simulink model "DNN_Final_Model"  (R2023a)
settings: Solver=VariableStepAuto  StartTime=0.0  StopTime=30  RelTol=1e-3
undefined symbols (not defined in the file or in its folder): c1, K1, k1, k2, m1, m2
libraries: simulink x5, spsVoltageMeasurementLib x3, slpidlib x2, eeGeneralControl x1, spsUniversalBridgeLib x1, spsDCVoltageSourceLib x1, sps_lib x1
settings Model: Creator=liu  LastModifiedBy=Probook
settings SolverCC: AlgebraicLoopSolver=TrustRegion
settings DataIOCC: ReturnWorkspaceOutputs=off
settings DebuggingCC: UnconnectedInputMsg=warning  UnconnectedOutputMsg=warning  UnconnectedLineMsg=warning  ArithmeticOperatorsInVariantConditions=warning
settings ModelReferenceCC: EnableRefExpFcnMdlSchedulingChecks=on
settings SFSimCC: CustomCodeUndefinedFunction=UseInterfaceOnly

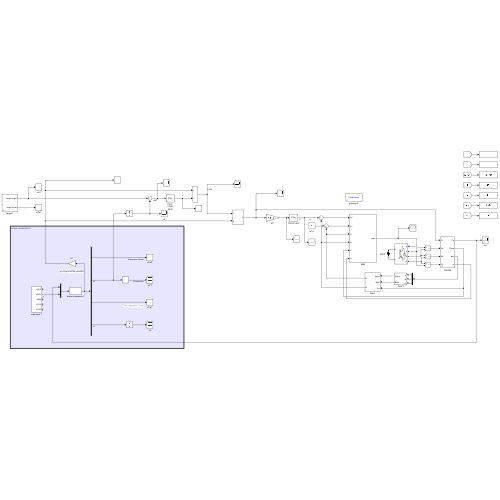
[thumbnail: Simulink's stored preview of the top-level diagram]
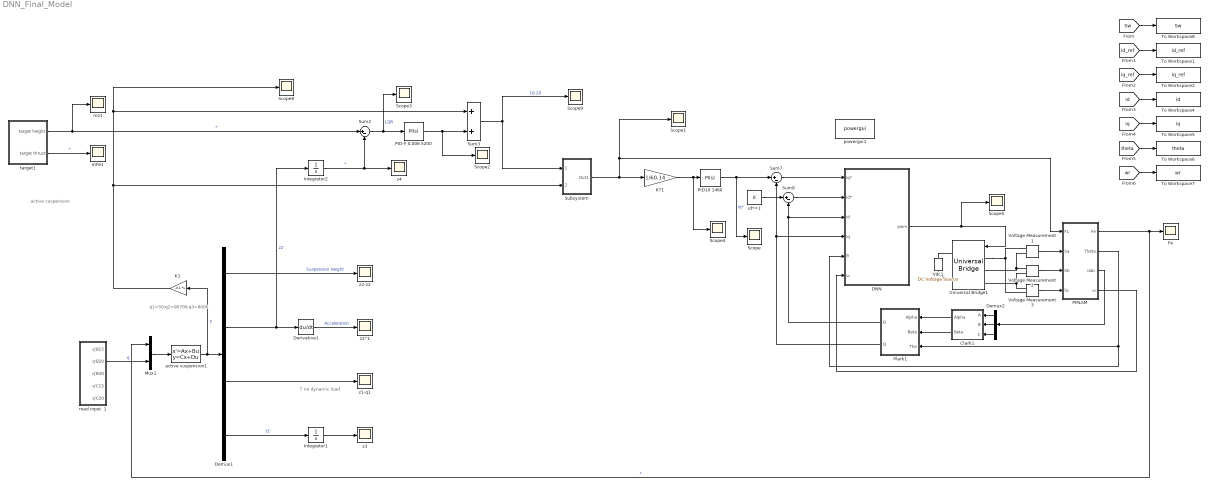
== system DNN_Final_Model ==
  note: T ire dynamic load
  note: active suspension
  note: q1=50;q2=90700;q3=8000
  Clark1 : Subsystem
  DNN : Subsystem
  Demux1 : Demux
  Demux2 : Demux  Outputs=3
  Derivative1 : Derivative
  Fe : Scope
  Integrator1 : Integrator
  Integrator2 : Integrator
  K1 : Gain  Gain=-K1  Multiplication=Matrix(K*u)
  KT1 : Gain  Gain=1/60.14
  Mux1 : Mux  Inputs=2
  PID-F 0.006 5200 : slpidlib/PID Controller  Controller=PI  Form=Parallel  TimeDomain=Continuous-time  UseExternalTs=off  SampleTime=-1  IntegratorMethod=Forward Euler  FilterMethod=Forward Euler  ControllerParametersSource=internal  P=0.006  I=62000  UseKiTs=off  D=10  N=100  UseFilter=on  TunerSelectOption=Transfer Function Based (PID Tuner App)  InitialConditionSource=internal  InitialConditionForIntegrator=0  InitialConditionForFilter=0  DifferentiatorICPrevScaledInput=0  ExternalReset=none  TrackingMode=off  Kt=1  LimitOutput=off  SatLimitsSource=internal  UpperSaturationLimit=inf  LowerSaturationLimit=-inf  LinearizeAsGain=on  AntiWindupMode=none  Kb=1  LimitIntegrator=off  UpperIntegratorSaturationLimit=inf  LowerIntegratorSaturationLimit=-inf  POutMin=[]  POutMax=[]  IOutMin=[]  IOutMax=[]  DOutMin=[]  DOutMax=[]  NOutMin=[]  NOutMax=[]  SumOutMin=[]  SumOutMax=[]  SaturationOutMin=[]  SaturationOutMax=[]  PParamMin=[]  PParamMax=[]  IParamMin=[]  IParamMax=[]  DParamMin=[]  DParamMax=[]  NParamMin=[]  NParamMax=[]  KbParamMin=[]  KbParamMax=[]  KtParamMin=[]  KtParamMax=[]  KbOutMin=[]  KbOutMax=[]  KtOutMin=[]  KtOutMax=[]  IntegratorOutMin=[]  IntegratorOutMax=[]  FilterOutMin=[]  FilterOutMax=[]  SumI1OutMin=[]  SumI1OutMax=[]  SumI2OutMin=[]  SumI2OutMax=[]  SumI3OutMin=[]  SumI3OutMax=[]  SumI4OutMin=[]  SumI4OutMax=[]  SumDOutMin=[]  SumDOutMax=[]  DifferentiatorOutMin=[]  DifferentiatorOutMax=[]  FilterDiffOutCoefMin=[]  FilterDiffOutCoefMax=[]  ReciprocalOutMin=[]  ReciprocalOutMax=[]  SumDenOutMin=[]  SumDenOutMax=[]  SumNumOutMin=[]  SumNumOutMax=[]  DivideOutMin=[]  DivideOutMax=[]  UdiffTsProdOutMin=[]  UdiffTsProdOutMax=[]  NTsProdOutMin=[]  NTsProdOutMax=[]  UintegralTsProdOutMin=[]  UintegralTsProdOutMax=[]  UngainTsProdOutMin=[]  UngainTsProdOutMax=[]  ClampingZeroOutDataTypeStr=Inherit: Inherit via back propagation  ClampingZeroOutMin=[]  ClampingZeroOutMax=[]  FilterDenConstantOutDataTypeStr=Inherit: Inherit via back propagation  FilterDenConstantOutMin=[]  FilterDenConstantOutMax=[]  PCopyOutDataTypeStr=Inherit: Inherit via back propagation  PCopyOutMin=[]  PCopyOutMax=[]  NCopyOutDataTypeStr=Inherit: Inherit via back propagation  NCopyOutMin=[]  NCopyOutMax=[]  IntegratorContinuousStateAttributes=''  IntegratorStateMustResolveToSignalObject=off  IntegratorRTWStateStorageClass=Auto  FilterContinuousStateAttributes=''  FilterStateMustResolveToSignalObject=off  FilterRTWStateStorageClass=Auto  ParallelPVariant=InternalParameters  IdealPVariant=Disabled  IVariant=InternalParameters  DVariant=Disabled  IntegratorVariant=Continuous  SatVariant=Disabled  AWVariant=Passthrough  PCopyVariant=Disabled  TRVariant=Disabled  FdbkBlocksVariant=Forward  IdealPFdbkVariant=Disabled  SatFdbkVariant=Disabled  DerivativeFilterVariant=Disabled  NVariant=Disabled  NCopyVariant=Disabled_SignalSpec  FilterICVariant=Disabled  IntegratorICVariant=InternalICs  ExternalResetVariant=Disabled  TRSumVariant=Passthrough  SumFdbkVariant=Disabled  SumVariant=Sum_PI  TsampFilterVariant=InternalTs  TsampNgainVariant=Passthrough  TsampIntegralVariant=Disabled_SignalSpec  ExternalSaturationOutDataTypeStr=Inherit: Same as second input
  PID10 1460 : slpidlib/PID Controller  Controller=PI  Form=Parallel  TimeDomain=Continuous-time  UseExternalTs=off  SampleTime=-1  IntegratorMethod=Forward Euler  FilterMethod=Forward Euler  ControllerParametersSource=internal  P=0.1  I=0.000001  UseKiTs=off  D=0  N=100  UseFilter=on  TunerSelectOption=Transfer Function Based (PID Tuner App)  InitialConditionSource=internal  InitialConditionForIntegrator=0  InitialConditionForFilter=0  DifferentiatorICPrevScaledInput=0  ExternalReset=none  TrackingMode=off  Kt=1  LimitOutput=off  SatLimitsSource=internal  UpperSaturationLimit=inf  LowerSaturationLimit=-inf  LinearizeAsGain=on  AntiWindupMode=none  Kb=1  LimitIntegrator=off  UpperIntegratorSaturationLimit=inf  LowerIntegratorSaturationLimit=-inf  POutMin=[]  POutMax=[]  IOutMin=[]  IOutMax=[]  DOutMin=[]  DOutMax=[]  NOutMin=[]  NOutMax=[]  SumOutMin=[]  SumOutMax=[]  SaturationOutMin=[]  SaturationOutMax=[]  PParamMin=[]  PParamMax=[]  IParamMin=[]  IParamMax=[]  DParamMin=[]  DParamMax=[]  NParamMin=[]  NParamMax=[]  KbParamMin=[]  KbParamMax=[]  KtParamMin=[]  KtParamMax=[]  KbOutMin=[]  KbOutMax=[]  KtOutMin=[]  KtOutMax=[]  IntegratorOutMin=[]  IntegratorOutMax=[]  FilterOutMin=[]  FilterOutMax=[]  SumI1OutMin=[]  SumI1OutMax=[]  SumI2OutMin=[]  SumI2OutMax=[]  SumI3OutMin=[]  SumI3OutMax=[]  SumI4OutMin=[]  SumI4OutMax=[]  SumDOutMin=[]  SumDOutMax=[]  DifferentiatorOutMin=[]  DifferentiatorOutMax=[]  FilterDiffOutCoefMin=[]  FilterDiffOutCoefMax=[]  ReciprocalOutMin=[]  ReciprocalOutMax=[]  SumDenOutMin=[]  SumDenOutMax=[]  SumNumOutMin=[]  SumNumOutMax=[]  DivideOutMin=[]  DivideOutMax=[]  UdiffTsProdOutMin=[]  UdiffTsProdOutMax=[]  NTsProdOutMin=[]  NTsProdOutMax=[]  UintegralTsProdOutMin=[]  UintegralTsProdOutMax=[]  UngainTsProdOutMin=[]  UngainTsProdOutMax=[]  ClampingZeroOutDataTypeStr=Inherit: Inherit via back propagation  ClampingZeroOutMin=[]  ClampingZeroOutMax=[]  FilterDenConstantOutDataTypeStr=Inherit: Inherit via back propagation  FilterDenConstantOutMin=[]  FilterDenConstantOutMax=[]  PCopyOutDataTypeStr=Inherit: Inherit via back propagation  PCopyOutMin=[]  PCopyOutMax=[]  NCopyOutDataTypeStr=Inherit: Inherit via back propagation  NCopyOutMin=[]  NCopyOutMax=[]  IntegratorContinuousStateAttributes=''  IntegratorStateMustResolveToSignalObject=off  IntegratorRTWStateStorageClass=Auto  FilterContinuousStateAttributes=''  FilterStateMustResolveToSignalObject=off  FilterRTWStateStorageClass=Auto  ParallelPVariant=InternalParameters  IdealPVariant=Disabled  IVariant=InternalParameters  DVariant=Disabled  IntegratorVariant=Continuous  SatVariant=Disabled  AWVariant=Passthrough  PCopyVariant=Disabled  TRVariant=Disabled  FdbkBlocksVariant=Forward  IdealPFdbkVariant=Disabled  SatFdbkVariant=Disabled  DerivativeFilterVariant=Disabled  NVariant=Disabled  NCopyVariant=Disabled_SignalSpec  FilterICVariant=Disabled  IntegratorICVariant=InternalICs  ExternalResetVariant=Disabled  TRSumVariant=Passthrough  SumFdbkVariant=Disabled  SumVariant=Sum_PI  TsampFilterVariant=InternalTs  TsampNgainVariant=Passthrough  TsampIntegralVariant=Disabled_SignalSpec  ExternalSaturationOutDataTypeStr=Inherit: Same as second input
  PMLSM : Subsystem  mask{Ld=0.0073, Lq=0.0073, M=10, B=0.8, R=1.5, tao=0.0077, np=16, flux=0.09}
      mask prompts: Ld "直轴电抗/H"; Lq "交轴电抗/H"; M "动子质量/kg"; B "粘滞摩擦系数/(N.s/m)"; R "电枢电阻/Ω"; tao "极距/m"; np "极对数"; flux "永磁磁链/Wb"
  Plark1 : Subsystem
  Scope{,1..5,8..9} (8 alike) : Scope
  Subsystem : Subsystem
  Sum2 : Sum  Inputs=|+-
  Sum3 : Sum
  Sum7 : Sum  Inputs=|+-
  Sum8 : Sum  Inputs=|+-
  To Workspace1 : ToWorkspace  VariableName=id_ref  SaveFormat=Structure With Time  SampleTime=-1
  To Workspace2 : ToWorkspace  VariableName=iq_ref  SaveFormat=Structure With Time  SampleTime=-1
  To Workspace4 : ToWorkspace  VariableName=id  SaveFormat=Structure With Time  SampleTime=-1
  To Workspace5 : ToWorkspace  VariableName=iq  SaveFormat=Structure With Time  SampleTime=-1
  To Workspace6 : ToWorkspace  VariableName=theta  SaveFormat=Structure With Time  SampleTime=-1
  To Workspace7 : ToWorkspace  VariableName=wr  SaveFormat=Structure With Time  SampleTime=-1
  To Workspace8 : ToWorkspace  VariableName=Sw  SaveFormat=Structure With Time  SampleTime=-1
  Universal Bridge1 : spsUniversalBridgeLib/Universal Bridge  Arms=3  SnubberResistance=1e5  SnubberCapacitance=inf  Device=IGBT / Diodes  Ron=1e-3  Lon=0  ForwardVoltages="[  0  0  ]"  ForwardVoltage=0  GTOparameters=[ 10e-6 , 20e-6 ]  IGBTparameters=[ 1e-6 , 2e-6 ]  Measurements=None  Measurements_2=None  converterType=Rectifier
  Vdc1 : spsDCVoltageSourceLib/DC Voltage Source  Amplitude=220  Measurements=None
  Voltage Measurement1 : spsVoltageMeasurementLib/Voltage Measurement  PhasorSimulation=off  OutputType=Complex  PSBequivalent=0
  Voltage Measurement2 : spsVoltageMeasurementLib/Voltage Measurement  PhasorSimulation=off  OutputType=Complex  PSBequivalent=0
  Voltage Measurement3 : spsVoltageMeasurementLib/Voltage Measurement  PhasorSimulation=off  OutputType=Complex  PSBequivalent=0
  active suspension1 : StateSpace  A=[0 1 0 -1;-k2/m2 -c1/m2 0 c1/m2;0 0 0 1;k2/m1 c1/m1 -k1/m1 -c1/m1]  B=[0 0;1/m2 0;0 -1;-1/m1 0]  C=[1 0 0 0;0 1 0 0;0 0 1 0;0 0 0 1]  D=[0 0;0 0;0 0;0 0]  InitialCondition=0
  id*=1 : Constant  Value=0
  mFe1 : Scope
  mz1 : Scope
  powergui1 : sps_lib/powergui  Priority=1  SimulationMode=Continuous  SampleTime=50e-6  frequency=60  Iterations=50  frequencyindice=0  Pbase=100e6  ErrMax=1e-4  UnitsV=kV  UnitsW=MW  buscounter=0  FunctionMessages=off  echomessages=off  EnableUseOfTLC=off  CurrentSourceSwitches=off  DisableSnubberDevices=off  DisableRonSwitches=off  DisableVfSwitches=off  DisplayEquations=off  AutomaticDiscreteSolvers=off  SolverType=Tustin/Backward Euler (TBE)  Interpol=off  ExternalGateDelay=off  methode=off  Ts=100  x0status=blocks  SPID=on  SwTol=0  HookPort=off  NonlinearTolerance=1e-4  nMaxIteration=100  ContinueOnMaxIteration=off  RestoreLinks=warning  ResistiveCurrentMeasurement=off  Frange=[0:2:500]  Ylog=off  Xlog=on  ShowGrid=off  save=off  variable=ZData  structure=0  ZoomFFT=off  StartTime=0.0  cycles=1  DisplayStyle=1  fundamental=60  FreqAxis=off  MaxFrequency=1000  frequencyindicesteady=1  RmsSteady=1  display=off
  road input  1 : Subsystem
  target1 : Subsystem  mask{x=0.08}
  z1-q1 : Scope
  z2''1 : Scope
  z2-z2 : Scope
  z3 : Scope
  z4 : Scope
  wires:
  Mux1/1 -> active suspension1/1
  active suspension1/1 -> Demux1/1, K1/1  "y"
  Demux1/3 -> z1-q1/1
  Integrator2/1 -> Sum2/2, z4/1  "*"
  K1/1 -> Scope8/1, Sum3/1, Subsystem/2(2)
  Integrator1/1 -> z3/1
  Demux1/1 -> z2-z2/1  "Suspension Height"
  PID-F 0.006 5200/1 -> Scope2/1, Sum3/2
  Demux1/2 -> Integrator2/1, Derivative1/1  "z2'"
  Sum2/1 -> Scope3/1, PID-F 0.006 5200/1  "LQR"
  Demux1/4 -> Integrator1/1  "z1'"
  Derivative1/1 -> z2''1/1  "Acceleration"
  target1/2(target thrust) -> mFe1/1  "*"
  target1/1(target height) -> mz1/1, Sum2/1  "*"
  Demux2/2 -> Clark1/2(B)
  Plark1/1(D) -> Sum8/2, DNN/3(id)
  Sum8/1 -> DNN/2(id*)
  Sum7/1 -> DNN/1(iq*)
  DNN/1(pwm) -> Scope5/1, Universal Bridge1/1
  PMLSM/3(iabc) -> Demux2/1
  Plark1/2(Q) -> DNN/4(iq), Sum7/2
  Voltage Measurement1/1 -> PMLSM/2(Sa)
  PMLSM/2(Theta) -> DNN/5(θ), Plark1/3(The)
  Demux2/3 -> Clark1/3(C)
  Demux2/1 -> Clark1/1(A)
  Voltage Measurement2/1 -> PMLSM/3(Sb)
  Clark1/2(Beta) -> Plark1/2(Beta)
  PMLSM/4(ω) -> DNN/6(ω)
  PMLSM/1(Fe) -> Mux1/1, Fe/1  "*"
  Clark1/1(Alpha) -> Plark1/1(Alpha)
  id*=1/1 -> Sum8/1
  PID10 1460/1 -> Scope/1, Sum7/1  "iq*"
  Voltage Measurement3/1 -> PMLSM/4(Sc)
  KT1/1 -> Scope4/1, PID10 1460/1
  road input  1/2("q'B20 ") -> Mux1/2  "q'"
  Sum3/1 -> Scope9/1, Subsystem/1(1)  "10-20"
  Subsystem/1(Out1) -> Scope1/1, PMLSM/1(FL), KT1/1
  [iq_ref] -> To Workspace2/1
  [iq] -> To Workspace5/1
  [wr] -> To Workspace7/1
  [id_ref] -> To Workspace1/1
  [id] -> To Workspace4/1
  [theta] -> To Workspace6/1
  [Sw] -> To Workspace8/1
  connections:
  Universal Bridge1/LConn1 -- Voltage Measurement3/LConn2 -- Voltage Measurement1/LConn1
  Voltage Measurement1/LConn2 -- Universal Bridge1/LConn2 -- Voltage Measurement2/LConn1
  Voltage Measurement2/LConn2 -- Voltage Measurement3/LConn1 -- Universal Bridge1/LConn3
  Universal Bridge1/RConn1 -- Vdc1/RConn1
  Universal Bridge1/RConn2 -- Vdc1/LConn1

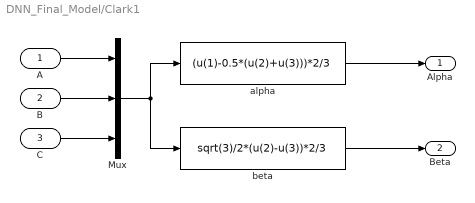
== system DNN_Final_Model/Clark1 ==
  A : Inport
  B : Inport  Port=2
  C : Inport  Port=3
  Mux : Mux  Inputs=3
  alpha : Fcn  Expr=(u(1)-0.5*(u(2)+u(3)))*2/3
  beta : Fcn  Expr=sqrt(3)/2*(u(2)-u(3))*2/3
  Alpha : Outport  VectorParamsAs1DForOutWhenUnconnected=off
  Beta : Outport  Port=2  VectorParamsAs1DForOutWhenUnconnected=off
  wires:
  alpha/1 -> Alpha/1
  B/1 -> Mux/2
  C/1 -> Mux/3
  A/1 -> Mux/1
  Mux/1 -> beta/1, alpha/1
  beta/1 -> Beta/1

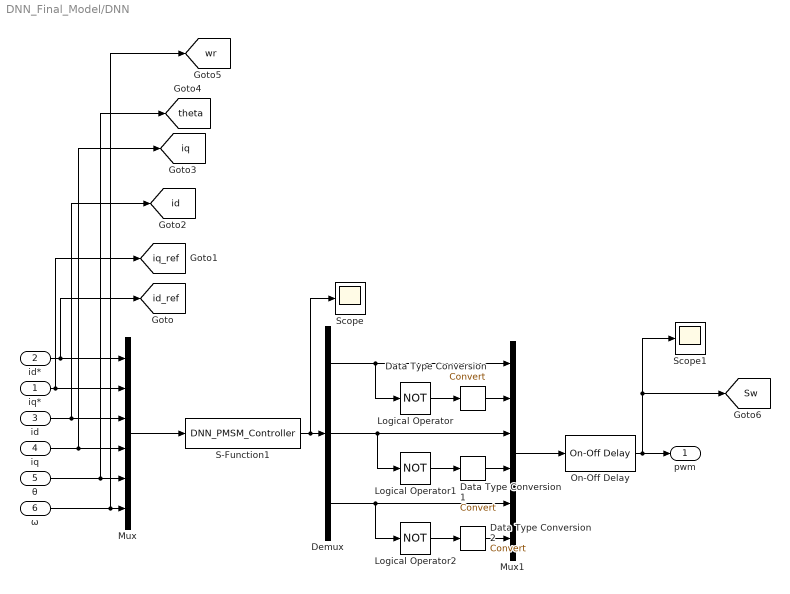
== system DNN_Final_Model/DNN ==
  iq* : Inport
  id* : Inport  Port=2
  id : Inport  Port=3
  iq : Inport  Port=4
  θ : Inport  Port=5
  ω : Inport  Port=6
  Data Type Conversion : DataTypeConversion  SaturateOnIntegerOverflow=off  RndMeth=Floor
  Data Type Conversion1 : DataTypeConversion  SaturateOnIntegerOverflow=off  RndMeth=Floor
  Data Type Conversion2 : DataTypeConversion  SaturateOnIntegerOverflow=off  RndMeth=Floor
  Demux : Demux  Outputs=3
  Logical Operator : Logic  Operator=NOT  AllPortsSameDT=off  OutDataTypeStr=boolean
  Logical Operator1 : Logic  Operator=NOT  AllPortsSameDT=off  OutDataTypeStr=boolean
  Logical Operator2 : Logic  Operator=NOT  AllPortsSameDT=off  OutDataTypeStr=boolean
  Mux : Mux  Inputs=6
  Mux1 : Mux  Inputs=6
  "On-Off Delay " : eeGeneralControl/On-Off Delay  LabelModeActiveChoice=Discrete  Td_on=1e-3  Td_off=0  IC=0  Ts=1e-3
  S-Function1 : S-Function  FunctionName=DNN_PMSM_Controller  SFunctionDeploymentMode=off  EnableBusSupport=off
  Scope : Scope
  Scope1 : Scope
  pwm : Outport  VectorParamsAs1DForOutWhenUnconnected=off
  tag scope: Sw=global, id=global, id_ref=global, iq=global, iq_ref=global, theta=global, wr=global
  wires:
  iq*/1 -> Mux/2, [iq_ref]
  ω/1 -> [wr], Mux/6
  id*/1 -> Mux/1, [id_ref]
  iq/1 -> Mux/4, [iq]
  θ/1 -> Mux/5, [theta]
  id/1 -> [id], Mux/3
  Mux/1 -> S-Function1/1
  "On-Off Delay "/1 -> pwm/1, Scope1/1, [Sw]
  Demux/2 -> Logical Operator1/1, Mux1/3
  Logical Operator1/1 -> Data Type Conversion1/1
  Logical Operator2/1 -> Data Type Conversion2/1
  Demux/3 -> Logical Operator2/1, Mux1/5
  Logical Operator/1 -> Data Type Conversion/1
  S-Function1/1 -> Scope/1, Demux/1
  Mux1/1 -> "On-Off Delay "/1
  Data Type Conversion1/1 -> Mux1/4
  Data Type Conversion2/1 -> Mux1/6
  Data Type Conversion/1 -> Mux1/2
  Demux/1 -> Logical Operator/1, Mux1/1

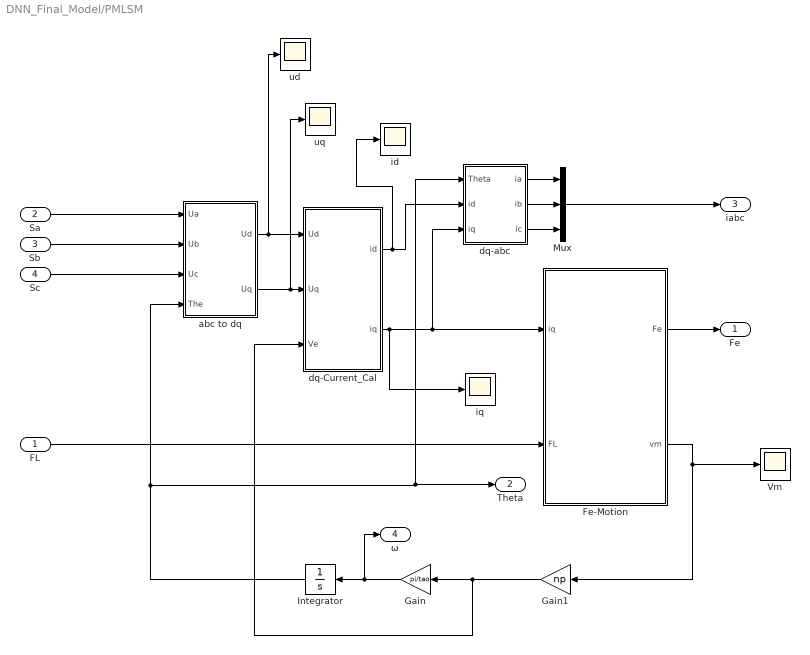
== system DNN_Final_Model/PMLSM ==
  FL : Inport
  Sa : Inport  Port=2
  Sb : Inport  Port=3
  Sc : Inport  Port=4
  Fe-Motion : Subsystem
  Gain : Gain  Gain=pi/tao
  Gain1 : Gain  Gain=np
  Integrator : Integrator
  Mux : Mux  Inputs=3
  Vm : Scope
  abc to dq : Subsystem
  dq-Current_Cal : Subsystem
  dq-abc : Subsystem
  id : Scope
  iq : Scope
  ud : Scope
  uq : Scope
  Fe : Outport  VectorParamsAs1DForOutWhenUnconnected=off
  Theta : Outport  Port=2  VectorParamsAs1DForOutWhenUnconnected=off
  iabc : Outport  Port=3  VectorParamsAs1DForOutWhenUnconnected=off
  ω : Outport  Port=4  VectorParamsAs1DForOutWhenUnconnected=off
  wires:
  Sb/1 -> abc to dq/2(Ub)
  Gain/1 -> ω/1, Integrator/1
  Gain1/1 -> Gain/1, dq-Current_Cal/3(Ve)
  dq-Current_Cal/2(iq) -> iq/1, Fe-Motion/1(iq), dq-abc/3(iq)
  abc to dq/1(Ud) -> dq-Current_Cal/1(Ud), ud/1
  Fe-Motion/1(Fe) -> Fe/1
  dq-abc/1(ia) -> Mux/1
  abc to dq/2(Uq) -> uq/1, dq-Current_Cal/2(Uq)
  FL/1 -> Fe-Motion/2(FL)
  Mux/1 -> iabc/1
  Integrator/1 -> abc to dq/4(The), Theta/1, dq-abc/1(Theta)
  Sc/1 -> abc to dq/3(Uc)
  dq-abc/2(ib) -> Mux/2
  dq-Current_Cal/1(id) -> id/1, dq-abc/2(id)
  Sa/1 -> abc to dq/1(Ua)
  dq-abc/3(ic) -> Mux/3
  Fe-Motion/2(vm) -> Vm/1, Gain1/1

== system DNN_Final_Model/Plark1 ==
  Alpha : Inport
  Beta : Inport  Port=2
  The : Inport  Port=3
  Mux : Mux  Inputs=3
  d : Fcn  Expr=u(1)*cos(u(3))+u(2)*sin(u(3))
  q : Fcn  Expr=-u(1)*sin(u(3))+u(2)*cos(u(3))
  D : Outport  VectorParamsAs1DForOutWhenUnconnected=off
  Q : Outport  Port=2  VectorParamsAs1DForOutWhenUnconnected=off
  wires:
  d/1 -> D/1
  Beta/1 -> Mux/2
  Alpha/1 -> Mux/1
  Mux/1 -> q/1, d/1
  q/1 -> Q/1
  The/1 -> Mux/3

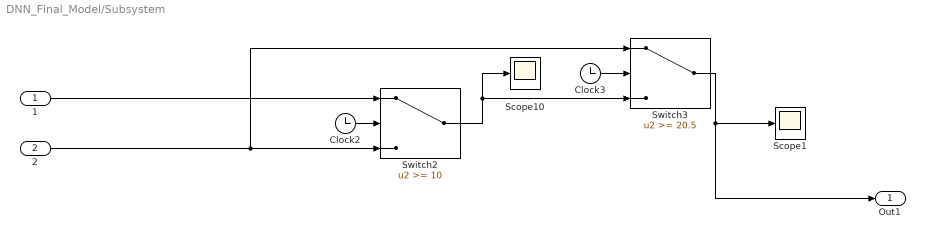
== system DNN_Final_Model/Subsystem ==
  1 : Inport
  2 : Inport  Port=2
  Clock2 : Clock
  Clock3 : Clock
  Scope1 : Scope
  Scope10 : Scope
  Switch2 : Switch  Threshold=10  ZeroCross=off  SaturateOnIntegerOverflow=off  InputSameDT=off
  Switch3 : Switch  Threshold=20.5  ZeroCross=off  SaturateOnIntegerOverflow=off  InputSameDT=off
  Out1 : Outport  VectorParamsAs1DForOutWhenUnconnected=off
  wires:
  Clock3/1 -> Switch3/2
  1/1 -> Switch2/1
  Switch3/1 -> Out1/1, Scope1/1
  Switch2/1 -> Scope10/1, Switch3/3
  2/1 -> Switch2/3, Switch3/1
  Clock2/1 -> Switch2/2

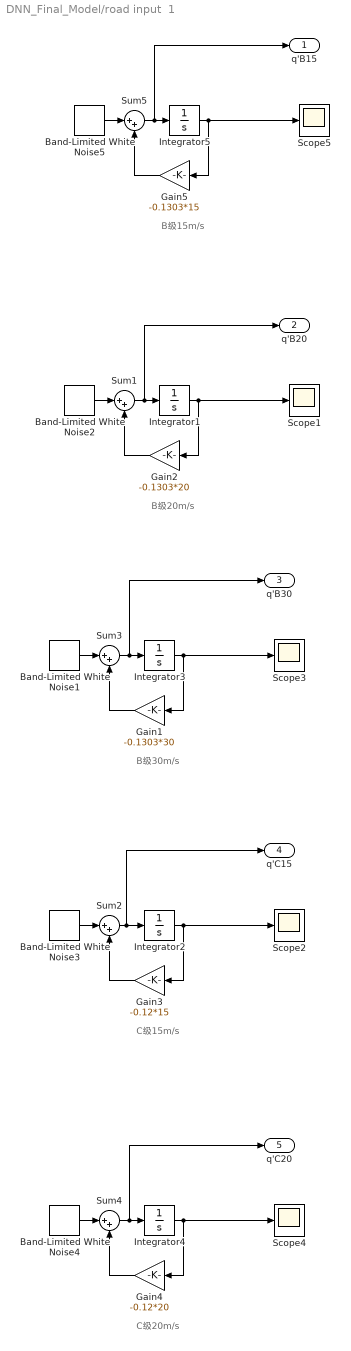
== system DNN_Final_Model/road input  1 ==
  note: B级20m/s
  note: B级30m/s
  note: C级20m/s
  note: C级15m/s
  note: B级15m/s
  Band-Limited White Noise1 : simulink/Sources/Band-Limited White Noise  Cov=[0.0007575]  Ts=0.01  seed=[23341]
  Band-Limited White Noise2 : simulink/Sources/Band-Limited White Noise  Cov=[0.000505]  Ts=0.01  seed=[23341]
  Band-Limited White Noise3 : simulink/Sources/Band-Limited White Noise  Cov=[0.00151]  Ts=0.01  seed=[23341]
  Band-Limited White Noise4 : simulink/Sources/Band-Limited White Noise  Cov=[0.00202]  Ts=0.01  seed=[23341]
  Band-Limited White Noise5 : simulink/Sources/Band-Limited White Noise  Cov=[0.0003788]  Ts=0.01  seed=[23341]
  Gain1 : Gain  Gain=-0.1303*30
  Gain2 : Gain  Gain=-0.1303*20
  Gain3 : Gain  Gain=-0.12*15
  Gain4 : Gain  Gain=-0.12*20
  Gain5 : Gain  Gain=-0.1303*15
  Integrator{1..5} (5 alike) : Integrator
  Scope{1..5} (5 alike) : Scope
  Sum{1..5} (5 alike) : Sum  Inputs=|++
  q'B15 : Outport  VectorParamsAs1DForOutWhenUnconnected=off
  "q'B20 " : Outport  Port=2  VectorParamsAs1DForOutWhenUnconnected=off
  q'B30 : Outport  Port=3  VectorParamsAs1DForOutWhenUnconnected=off
  q'C15 : Outport  Port=4  VectorParamsAs1DForOutWhenUnconnected=off
  q'C20 : Outport  Port=5  VectorParamsAs1DForOutWhenUnconnected=off
  wires:
  Sum1/1 -> "q'B20 "/1, Integrator1/1
  Band-Limited White Noise2/1 -> Sum1/1
  Integrator1/1 -> Scope1/1, Gain2/1
  Gain2/1 -> Sum1/2
  Gain4/1 -> Sum4/2
  Band-Limited White Noise4/1 -> Sum4/1
  Sum3/1 -> q'B30/1, Integrator3/1
  Integrator4/1 -> Scope4/1, Gain4/1
  Sum4/1 -> q'C20/1, Integrator4/1
  Band-Limited White Noise1/1 -> Sum3/1
  Integrator3/1 -> Scope3/1, Gain1/1
  Gain1/1 -> Sum3/2
  Band-Limited White Noise3/1 -> Sum2/1
  Gain3/1 -> Sum2/2
  Sum2/1 -> q'C15/1, Integrator2/1
  Integrator2/1 -> Scope2/1, Gain3/1
  Band-Limited White Noise5/1 -> Sum5/1
  Integrator5/1 -> Scope5/1, Gain5/1
  Sum5/1 -> q'B15/1, Integrator5/1
  Gain5/1 -> Sum5/2

== system DNN_Final_Model/target1 ==
  target valueFe : Subsystem
  targetz : Subsystem
  target height : Outport  VectorParamsAs1DForOutWhenUnconnected=off
  target thrust : Outport  Port=2  VectorParamsAs1DForOutWhenUnconnected=off
  wires:
  targetz/1(x*) -> target height/1
  targetz/2(Out1) -> target valueFe/1(In1)
  target valueFe/1(x*) -> target thrust/1

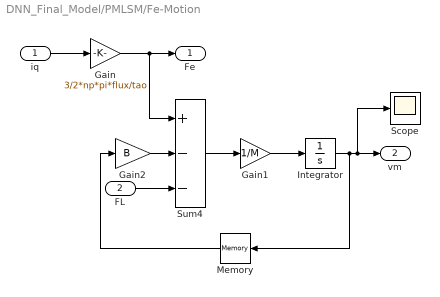
== system DNN_Final_Model/PMLSM/Fe-Motion ==
  iq : Inport
  FL : Inport  Port=2
  Gain : Gain  Gain=3/2*np*pi*flux/tao
  Gain1 : Gain  Gain=1/M
  Gain2 : Gain  Gain=B
  Integrator : Integrator
  Memory : Memory
  Scope : Scope
  Sum4 : Sum  Inputs=+--  SaturateOnIntegerOverflow=on
  Fe : Outport  VectorParamsAs1DForOutWhenUnconnected=off
  vm : Outport  Port=2  VectorParamsAs1DForOutWhenUnconnected=off
  wires:
  iq/1 -> Gain/1
  Gain/1 -> Sum4/1, Fe/1
  Sum4/1 -> Gain1/1
  FL/1 -> Sum4/3
  Gain1/1 -> Integrator/1
  Integrator/1 -> Memory/1, Scope/1, vm/1
  Gain2/1 -> Sum4/2
  Memory/1 -> Gain2/1

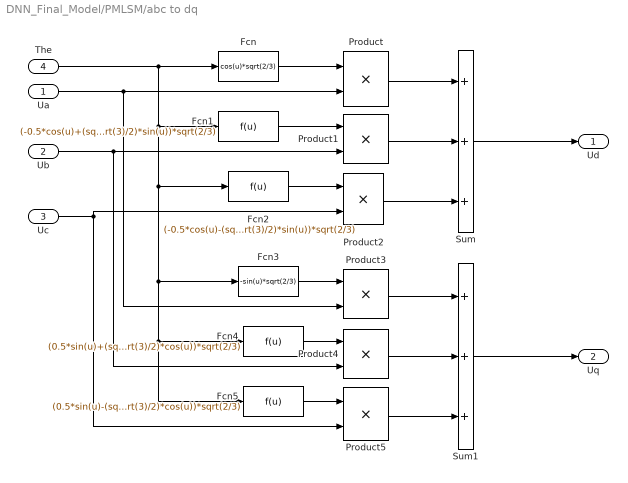
== system DNN_Final_Model/PMLSM/abc to dq ==
  Ua : Inport
  Ub : Inport  Port=2
  Uc : Inport  Port=3
  The : Inport  Port=4
  Fcn : Fcn  Expr=cos(u)*sqrt(2/3)
  Fcn1 : Fcn  Expr=(-0.5*cos(u)+(sqrt(3)/2)*sin(u))*sqrt(2/3)
  Fcn2 : Fcn  Expr=(-0.5*cos(u)-(sqrt(3)/2)*sin(u))*sqrt(2/3)
  Fcn3 : Fcn  Expr=-sin(u)*sqrt(2/3)
  Fcn4 : Fcn  Expr=(0.5*sin(u)+(sqrt(3)/2)*cos(u))*sqrt(2/3)
  Fcn5 : Fcn  Expr=(0.5*sin(u)-(sqrt(3)/2)*cos(u))*sqrt(2/3)
  Product{,1..5} (6 alike) : Product  SaturateOnIntegerOverflow=on  OutDataTypeStr=Inherit: Same as first input
  Sum : Sum  Inputs=+++  SaturateOnIntegerOverflow=on
  Sum1 : Sum  Inputs=+++  SaturateOnIntegerOverflow=on
  Ud : Outport  VectorParamsAs1DForOutWhenUnconnected=off
  Uq : Outport  Port=2  VectorParamsAs1DForOutWhenUnconnected=off
  wires:
  Product/1 -> Sum/1
  Product1/1 -> Sum/2
  Product4/1 -> Sum1/2
  Product5/1 -> Sum1/3
  Sum/1 -> Ud/1
  Fcn/1 -> Product/1
  The/1 -> Fcn1/1, Fcn3/1, Fcn5/1, Fcn4/1, Fcn2/1, Fcn/1
  Ua/1 -> Product/2, Product3/2
  Fcn1/1 -> Product1/1
  Ub/1 -> Product1/2, Product4/2
  Product2/1 -> Sum/3
  Uc/1 -> Product2/2, Product5/2
  Fcn2/1 -> Product2/1
  Sum1/1 -> Uq/1
  Product3/1 -> Sum1/1
  Fcn3/1 -> Product3/1
  Fcn4/1 -> Product4/1
  Fcn5/1 -> Product5/1

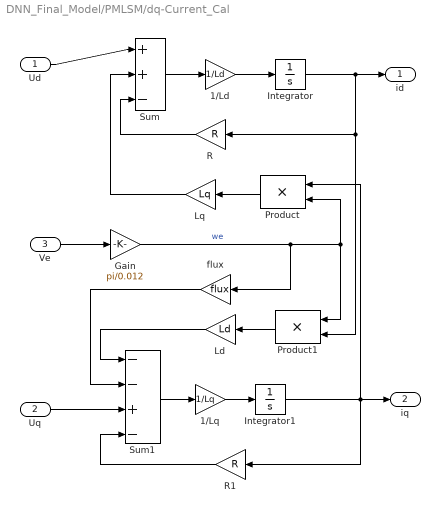
== system DNN_Final_Model/PMLSM/dq-Current_Cal ==
  Ud : Inport
  Uq : Inport  Port=2
  Ve : Inport  Port=3
  1/Ld : Gain  Gain=1/Ld  SaturateOnIntegerOverflow=on  OutDataTypeStr=Inherit: Same as input  ParamDataTypeStr=Inherit: Same as input
  1/Lq : Gain  Gain=1/Lq  SaturateOnIntegerOverflow=on  OutDataTypeStr=Inherit: Same as input  ParamDataTypeStr=Inherit: Same as input
  Gain : Gain  Gain=pi/0.012
  Integrator : Integrator  InitialCondition=0.01
  Integrator1 : Integrator
  Ld : Gain  Gain=Ld  SaturateOnIntegerOverflow=on  OutDataTypeStr=Inherit: Same as input  ParamDataTypeStr=Inherit: Same as input
  Lq : Gain  Gain=Lq  SaturateOnIntegerOverflow=on  OutDataTypeStr=Inherit: Same as input  ParamDataTypeStr=Inherit: Same as input
  Product : Product  SaturateOnIntegerOverflow=on  OutDataTypeStr=Inherit: Same as first input
  Product1 : Product  SaturateOnIntegerOverflow=on  OutDataTypeStr=Inherit: Same as first input
  R : Gain  Gain=R  SaturateOnIntegerOverflow=on  OutDataTypeStr=Inherit: Same as input  ParamDataTypeStr=Inherit: Same as input
  R1 : Gain  Gain=R  SaturateOnIntegerOverflow=on  OutDataTypeStr=Inherit: Same as input  ParamDataTypeStr=Inherit: Same as input
  Sum : Sum  Inputs=|++-  SaturateOnIntegerOverflow=on
  Sum1 : Sum  Inputs=--+-  SaturateOnIntegerOverflow=on
  flux : Gain  Gain=flux  SaturateOnIntegerOverflow=on  OutDataTypeStr=Inherit: Same as input  ParamDataTypeStr=Inherit: Same as input
  id : Outport  VectorParamsAs1DForOutWhenUnconnected=off
  iq : Outport  Port=2  VectorParamsAs1DForOutWhenUnconnected=off
  wires:
  Ud/1 -> Sum/1
  Sum/1 -> 1/Ld/1
  1/Ld/1 -> Integrator/1
  Integrator/1 -> Product1/2, R/1, id/1
  Product/1 -> Lq/1
  Lq/1 -> Sum/2
  Ve/1 -> Gain/1
  R/1 -> Sum/3
  R1/1 -> Sum1/4
  1/Lq/1 -> Integrator1/1
  Sum1/1 -> 1/Lq/1
  Integrator1/1 -> R1/1, Product/1, iq/1
  Product1/1 -> Ld/1
  Ld/1 -> Sum1/1
  Uq/1 -> Sum1/3
  flux/1 -> Sum1/2
  Gain/1 -> Product/2, Product1/1, flux/1  "we"

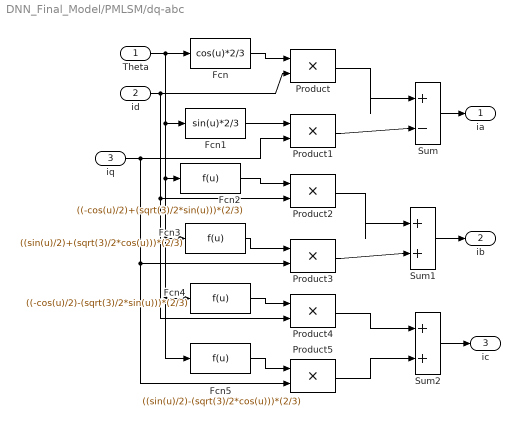
== system DNN_Final_Model/PMLSM/dq-abc ==
  Theta : Inport
  id : Inport  Port=2
  iq : Inport  Port=3
  Fcn : Fcn  Expr=cos(u)*2/3
  Fcn1 : Fcn  Expr=sin(u)*2/3
  Fcn2 : Fcn  Expr=((-cos(u)/2)+(sqrt(3)/2*sin(u)))*(2/3)
  Fcn3 : Fcn  Expr=((sin(u)/2)+(sqrt(3)/2*cos(u)))*(2/3)
  Fcn4 : Fcn  Expr=((-cos(u)/2)-(sqrt(3)/2*sin(u)))*(2/3)
  Fcn5 : Fcn  Expr=((sin(u)/2)-(sqrt(3)/2*cos(u)))*(2/3)
  Product{,1..5} (6 alike) : Product  SaturateOnIntegerOverflow=on  OutDataTypeStr=Inherit: Same as first input
  Sum : Sum  Inputs=|+-  SaturateOnIntegerOverflow=on
  Sum1 : Sum  Inputs=|++  SaturateOnIntegerOverflow=on
  Sum2 : Sum  SaturateOnIntegerOverflow=on
  ia : Outport  VectorParamsAs1DForOutWhenUnconnected=off
  ib : Outport  Port=2  VectorParamsAs1DForOutWhenUnconnected=off
  ic : Outport  Port=3  VectorParamsAs1DForOutWhenUnconnected=off
  wires:
  Fcn/1 -> Product/1
  Theta/1 -> Fcn5/1, Fcn4/1, Fcn3/1, Fcn2/1, Fcn1/1, Fcn/1
  id/1 -> Product4/2, Product2/2, Product/2
  Product/1 -> Sum/1
  Fcn1/1 -> Product1/1
  Product1/1 -> Sum/2
  iq/1 -> Product3/2, Product5/2, Product1/2
  Sum/1 -> ia/1
  Fcn2/1 -> Product2/1
  Fcn3/1 -> Product3/1
  Fcn5/1 -> Product5/1
  Fcn4/1 -> Product4/1
  Product2/1 -> Sum1/1
  Product3/1 -> Sum1/2
  Product4/1 -> Sum2/1
  Product5/1 -> Sum2/2
  Sum2/1 -> ic/1
  Sum1/1 -> ib/1

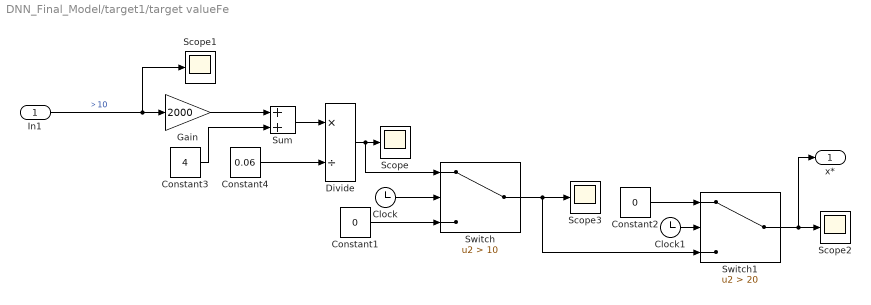
== system DNN_Final_Model/target1/target valueFe ==
  In1 : Inport
  Clock : Clock
  Clock1 : Clock
  Constant1 : Constant  Value=0
  Constant2 : Constant  Value=0
  Constant3 : Constant  Value=4
  Constant4 : Constant  Value=0.06
  Divide : Product  Inputs=*/
  Gain : Gain  Gain=2000
  Scope{,1..3} (4 alike) : Scope
  Sum : Sum
  Switch : Switch  Criteria=u2 > Threshold  Threshold=10  SaturateOnIntegerOverflow=off  InputSameDT=off
  Switch1 : Switch  Criteria=u2 > Threshold  Threshold=20  SaturateOnIntegerOverflow=off  InputSameDT=off
  x* : Outport  VectorParamsAs1DForOutWhenUnconnected=off
  wires:
  Gain/1 -> Sum/1
  Constant3/1 -> Sum/2
  Sum/1 -> Divide/1
  Constant4/1 -> Divide/2
  Clock/1 -> Switch/2
  Clock1/1 -> Switch1/2
  Switch/1 -> Switch1/3, Scope3/1
  Constant2/1 -> Switch1/1
  Constant1/1 -> Switch/3
  Switch1/1 -> x*/1, Scope2/1
  In1/1 -> Scope1/1, Gain/1  "＞10"
  Divide/1 -> Switch/1, Scope/1

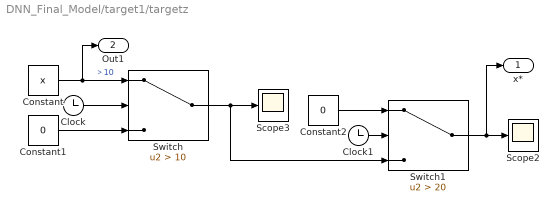
== system DNN_Final_Model/target1/targetz ==
  Clock : Clock
  Clock1 : Clock
  Constant : Constant  Value=x
  Constant1 : Constant  Value=0
  Constant2 : Constant  Value=0
  Scope2 : Scope
  Scope3 : Scope
  Switch : Switch  Criteria=u2 > Threshold  Threshold=10  SaturateOnIntegerOverflow=off  InputSameDT=off
  Switch1 : Switch  Criteria=u2 > Threshold  Threshold=20  SaturateOnIntegerOverflow=off  InputSameDT=off
  x* : Outport  VectorParamsAs1DForOutWhenUnconnected=off
  Out1 : Outport  Port=2  VectorParamsAs1DForOutWhenUnconnected=off
  wires:
  Switch1/1 -> x*/1, Scope2/1
  Constant1/1 -> Switch/3
  Constant2/1 -> Switch1/1
  Constant/1 -> Out1/1, Switch/1  "＞10"
  Switch/1 -> Switch1/3, Scope3/1
  Clock/1 -> Switch/2
  Clock1/1 -> Switch1/2
